simulink model "Temperature_Change_In_The_Water_Tank"  (R2024b)
settings: Solver=VariableStepAuto  StartTime=0.0  StopTime=10  RelTol=1e-3
settings Model: Creator=ksamb  LastModifiedBy=suman

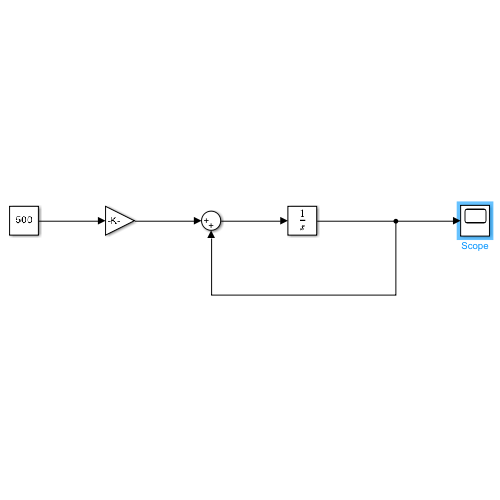
[thumbnail: Simulink's stored preview of the top-level diagram]
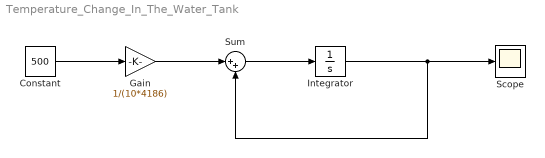
== system Temperature_Change_In_The_Water_Tank ==
  Constant : Constant  Value=500
  Gain : Gain  Gain=1/(10*4186)
  Integrator : Integrator  InitialCondition=20
  Scope : Scope
  Sum : Sum  Inputs=|++
  wires:
  Constant/1 -> Gain/1
  Sum/1 -> Integrator/1
  Integrator/1 -> Sum/2, Scope/1
  Gain/1 -> Sum/1
